simulink library "Teleop_lib"  (R2023b)
settings: Solver=VariableStepAuto  StartTime=0.0  StopTime=10.0  RelTol=1e-3
undefined symbols (not defined in the file): Spline_Num_Poses_default, Spline_Ref_Poses_default, TEST_Swerve_Mode_Override_Flag, TEST_Swerve_Mode_Steering, TEST_Swerve_Mode_Translation
settings Model: Creator=FIRSTMentor  LastModifiedBy=ander

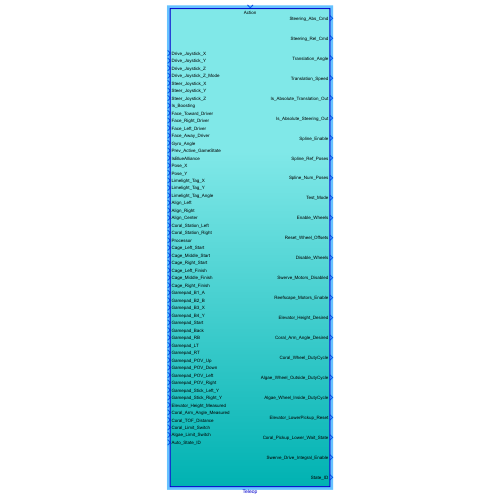
[thumbnail: Simulink's stored preview of the top-level diagram]
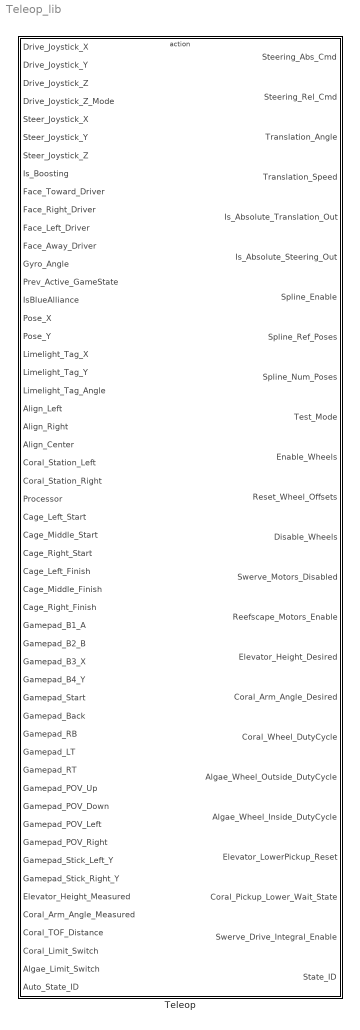
== system Teleop_lib ==
  Teleop : Subsystem  TreatAsAtomicUnit=on

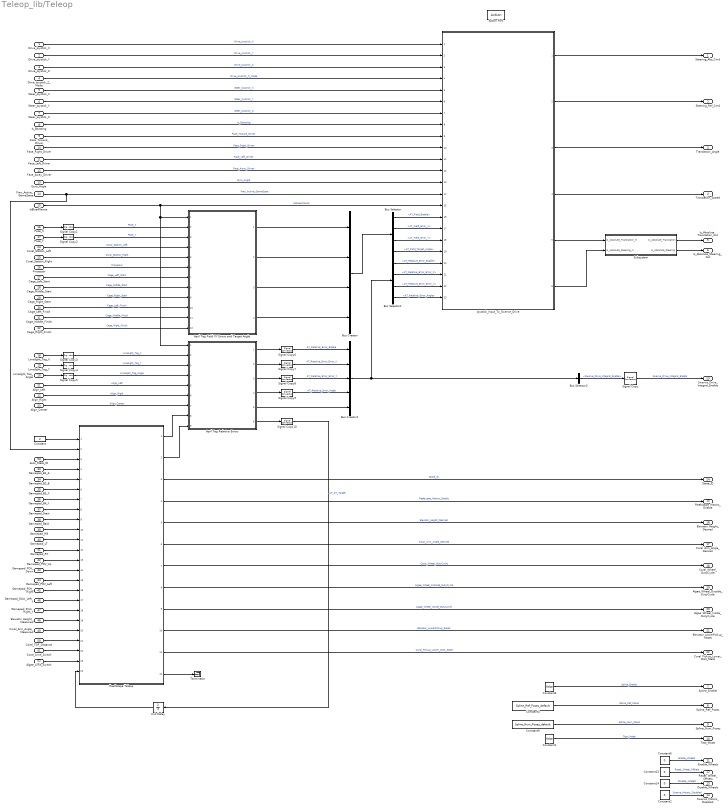
== system Teleop_lib/Teleop ==
  Drive_Joystick_X : Inport
  Drive_Joystick_Y : Inport  Port=2
  Drive_Joystick_Z : Inport  Port=3
  Drive_Joystick_Z_Mode : Inport  Port=4
  Steer_Joystick_X : Inport  Port=5
  Steer_Joystick_Y : Inport  Port=6
  Steer_Joystick_Z : Inport  Port=7
  Is_Boosting : Inport  Port=8
  Face_Toward_Driver : Inport  Port=9
  Face_Right_Driver : Inport  Port=10
  Face_Left_Driver : Inport  Port=11
  Face_Away_Driver : Inport  Port=12
  Gyro_Angle : Inport  Port=13
  Prev_Active_GameState : Inport  Port=14
  IsBlueAlliance : Inport  Port=15
  Pose_X : Inport  Port=16
  Pose_Y : Inport  Port=17
  Limelight_Tag_X : Inport  Port=18
  Limelight_Tag_Y : Inport  Port=19
  Limelight_Tag_Angle : Inport  Port=20
  Align_Left : Inport  Port=21
  Align_Right : Inport  Port=22
  Align_Center : Inport  Port=23
  Coral_Station_Left : Inport  Port=24
  Coral_Station_Right : Inport  Port=25
  Processor : Inport  Port=26
  Cage_Left_Start : Inport  Port=27
  Cage_Middle_Start : Inport  Port=28
  Cage_Right_Start : Inport  Port=29
  Cage_Left_Finish : Inport  Port=30
  Cage_Middle_Finish : Inport  Port=31
  Cage_Right_Finish : Inport  Port=32
  Gamepad_B1_A : Inport  Port=33
  Gamepad_B2_B : Inport  Port=34
  Gamepad_B3_X : Inport  Port=35
  Gamepad_B4_Y : Inport  Port=36
  Gamepad_Start : Inport  Port=37
  Gamepad_Back : Inport  Port=38
  Gamepad_RB : Inport  Port=39
  Gamepad_LT : Inport  Port=40
  Gamepad_RT : Inport  Port=41
  Gamepad_POV_Up : Inport  Port=42
  Gamepad_POV_Down : Inport  Port=43
  Gamepad_POV_Left : Inport  Port=44
  Gamepad_POV_Right : Inport  Port=45
  Gamepad_Stick_Left_Y : Inport  Port=46
  Gamepad_Stick_Right_Y : Inport  Port=47
  Elevator_Height_Measured : Inport  Port=48
  Coral_Arm_Angle_Measured : Inport  Port=49
  Coral_TOF_Distance : Inport  Port=50
  Coral_Limit_Switch : Inport  Port=51
  Algae_Limit_Switch : Inport  Port=52
  Auto_State_ID : Inport  Port=53
  Action Port : ActionPort  InitializeStates=reset
  April Tag Field XY Errors and Target Angle : Subsystem  ReferencedSubsystem=April_Tag_Field_Errors
  April Tag Relative Errors : Subsystem  ReferencedSubsystem=April_Tag_Relative_Errors
  Bus Creator : BusCreator  Inputs=4
  Bus Creator1 : BusCreator  Inputs=5
  Bus Selector : BusSelector  OutputSignals=AT_Field_Enable,AT_Field_Error_X,AT_Field_Error_Y,AT_Field_Target_Angle
  Bus Selector1 : BusSelector  OutputSignals=AT_Relative_Error_Enable,AT_Relative_Error_Error_X,AT_Relative_Error_Error_Y,AT_Relative_Error_Angle
  Bus Selector2 : BusSelector  OutputSignals=Swerve_Drive_Integral_Enable
  Constant : Constant  Value=2  OutDataTypeStr=uint8
  Constant1 : Constant  Value=false  OutDataTypeStr=boolean
  Constant13 : Constant  Value=0
  Constant14 : Constant  Value=0
  Constant2 : Constant  Value=0  OutDataTypeStr=boolean
  Constant3 : Constant  Value=false  OutDataTypeStr=boolean
  Constant4 : Constant  Value=Spline_Ref_Poses_default
  Constant6 : Constant  Value=0
  Constant9 : Constant  Value=Spline_Num_Poses_default  OutDataTypeStr=double
  Joystick_Input_To_Swerve_Drive : Subsystem  ReferencedSubsystem=Joystick_Input_To_Swerve_Drive_sub
  Reefscape Teleop : Subsystem  ReferencedSubsystem=Reefscape_Teleop_sub
  Signal Copy{,1..10} (11 alike) : SignalConversion  OverrideOpt=off
  Subsystem : Subsystem
  Terminator : Terminator
  Unit Delay : UnitDelay  SampleTime=-1  HasFrameUpgradeWarning=on
  Steering_Abs_Cmd : Outport
  Steering_Rel_Cmd : Outport  Port=2
  Translation_Angle : Outport  Port=3
  Translation_Speed : Outport  Port=4
  Is_Absolute_Translation_Out : Outport  Port=5
  Is_Absolute_Steering_Out : Outport  Port=6
  Spline_Enable : Outport  Port=7
  Spline_Ref_Poses : Outport  Port=8
  Spline_Num_Poses : Outport  Port=9
  Test_Mode : Outport  Port=10
  Enable_Wheels : Outport  Port=11
  Reset_Wheel_Offsets : Outport  Port=12
  Disable_Wheels : Outport  Port=13
  Swerve_Motors_Disabled : Outport  Port=14
  Reefscape_Motors_Enable : Outport  Port=15
  Elevator_Height_Desired : Outport  Port=16
  Coral_Arm_Angle_Desired : Outport  Port=17
  Coral_Wheel_DutyCycle : Outport  Port=18
  Algae_Wheel_Outside_DutyCycle : Outport  Port=19
  Algae_Wheel_Inside_DutyCycle : Outport  Port=20
  Elevator_LowerPickup_Reset : Outport  Port=21
  Coral_Pickup_Lower_Wait_State : Outport  Port=22
  Swerve_Drive_Integral_Enable : Outport  Port=23
  State_ID : Outport  Port=24
  wires:
  Signal Copy/1 -> Swerve_Drive_Integral_Enable/1  "Swerve_Drive_Integral_Enable"
  Steer_Joystick_X/1 -> Joystick_Input_To_Swerve_Drive/5  "Steer_Joystick_X"
  Steer_Joystick_Y/1 -> Joystick_Input_To_Swerve_Drive/6  "Steer_Joystick_Y"
  Drive_Joystick_X/1 -> Joystick_Input_To_Swerve_Drive/1  "Drive_Joystick_X"
  Drive_Joystick_Y/1 -> Joystick_Input_To_Swerve_Drive/2  "Drive_Joystick_Y"
  Joystick_Input_To_Swerve_Drive/1 -> Steering_Abs_Cmd/1
  Joystick_Input_To_Swerve_Drive/2 -> Steering_Rel_Cmd/1
  Joystick_Input_To_Swerve_Drive/3 -> Translation_Angle/1
  Joystick_Input_To_Swerve_Drive/4 -> Translation_Speed/1
  Is_Boosting/1 -> Joystick_Input_To_Swerve_Drive/8  "Is_Boosting"
  Constant9/1 -> Spline_Num_Poses/1  "Spline_Num_Poses"
  Constant4/1 -> Spline_Ref_Poses/1  "Spline_Ref_Poses"
  Constant3/1 -> Spline_Enable/1  "Spline_Enable"
  Constant1/1 -> Test_Mode/1  "Test_Mode"
  Drive_Joystick_Z/1 -> Joystick_Input_To_Swerve_Drive/3  "Drive_Joystick_Z"
  Steer_Joystick_Z/1 -> Joystick_Input_To_Swerve_Drive/7  "Steer_Joystick_Z"
  Face_Toward_Driver/1 -> Joystick_Input_To_Swerve_Drive/9  "Face_Toward_Driver"
  Face_Right_Driver/1 -> Joystick_Input_To_Swerve_Drive/10  "Face_Right_Driver"
  Face_Left_Driver/1 -> Joystick_Input_To_Swerve_Drive/11  "Face_Left_Driver"
  Face_Away_Driver/1 -> Joystick_Input_To_Swerve_Drive/12  "Face_Away_Driver"
  Pose_X/1 -> Signal Copy1/1
  Pose_Y/1 -> Signal Copy2/1
  IsBlueAlliance/1 -> Joystick_Input_To_Swerve_Drive/15, April Tag Relative Errors/1, April Tag Field XY Errors and Target Angle/1  "IsBlueAlliance"
  Drive_Joystick_Z_Mode/1 -> Joystick_Input_To_Swerve_Drive/4  "Drive_Joystick_Z_Mode"
  Gyro_Angle/1 -> Joystick_Input_To_Swerve_Drive/13  "Gyro_Angle"
  Align_Left/1 -> April Tag Relative Errors/5  "Align_Left"
  Align_Right/1 -> April Tag Relative Errors/6  "Align_Right"
  Align_Center/1 -> April Tag Relative Errors/7  "Align_Center"
  Limelight_Tag_X/1 -> Signal Copy3/1
  Limelight_Tag_Y/1 -> Signal Copy4/1
  Limelight_Tag_Angle/1 -> Signal Copy5/1
  Constant13/1 -> Reset_Wheel_Offsets/1  "Reset_Wheel_Offsets"
  Constant14/1 -> Disable_Wheels/1  "Disable_Wheels"
  Prev_Active_GameState/1 -> Joystick_Input_To_Swerve_Drive/14, Reefscape Teleop/2  "Prev_Active_GameState"
  Constant2/1 -> Swerve_Motors_Disabled/1  "Swerve_Motors_Disabled"
  Constant6/1 -> Enable_Wheels/1  "Enable_Wheels"
  Signal Copy3/1 -> April Tag Relative Errors/2  "Limelight_Tag_X"
  Signal Copy4/1 -> April Tag Relative Errors/3  "Limelight_Tag_Y"
  Signal Copy5/1 -> April Tag Relative Errors/4  "Limelight_Tag_Angle"
  Coral_Station_Left/1 -> April Tag Field XY Errors and Target Angle/4  "Coral_Station_Left"
  Coral_Station_Right/1 -> April Tag Field XY Errors and Target Angle/5  "Coral_Station_Right"
  Processor/1 -> April Tag Field XY Errors and Target Angle/6  "Processor"
  Signal Copy1/1 -> April Tag Field XY Errors and Target Angle/2  "Pose_X"
  Signal Copy2/1 -> April Tag Field XY Errors and Target Angle/3  "Pose_Y"
  Joystick_Input_To_Swerve_Drive/5 -> Subsystem/1(Is_Absolute_Translation_In)
  Joystick_Input_To_Swerve_Drive/6 -> Subsystem/2(Is_Absolute_Steering_In)
  Subsystem/1(Is_Absolute_Translation) -> Is_Absolute_Translation_Out/1
  Subsystem/2(Is_Absolute_Steering) -> Is_Absolute_Steering_Out/1
  Reefscape Teleop/1 -> April Tag Relative Errors/8
  April Tag Field XY Errors and Target Angle/1 -> Bus Creator/1
  April Tag Field XY Errors and Target Angle/2 -> Bus Creator/2
  April Tag Field XY Errors and Target Angle/3 -> Bus Creator/3
  April Tag Field XY Errors and Target Angle/4 -> Bus Creator/4
  April Tag Relative Errors/1 -> Signal Copy6/1
  April Tag Relative Errors/2 -> Signal Copy7/1
  April Tag Relative Errors/3 -> Signal Copy8/1
  April Tag Relative Errors/4 -> Signal Copy9/1
  Bus Creator/1 -> Bus Selector/1
  Bus Selector/1 -> Joystick_Input_To_Swerve_Drive/16  "<AT_Field_Enable>"
  Bus Selector/2 -> Joystick_Input_To_Swerve_Drive/17  "<AT_Field_Error_X>"
  Bus Selector/3 -> Joystick_Input_To_Swerve_Drive/18  "<AT_Field_Error_Y>"
  Bus Selector/4 -> Joystick_Input_To_Swerve_Drive/19  "<AT_Field_Target_Angle>"
  Bus Creator1/1 -> Bus Selector2/1, Bus Selector1/1
  Bus Selector1/1 -> Joystick_Input_To_Swerve_Drive/20  "<AT_Relative_Error_Enable>"
  Bus Selector1/2 -> Joystick_Input_To_Swerve_Drive/21  "<AT_Relative_Error_Error_X>"
  Bus Selector1/3 -> Joystick_Input_To_Swerve_Drive/22  "<AT_Relative_Error_Error_Y>"
  Bus Selector1/4 -> Joystick_Input_To_Swerve_Drive/23  "<AT_Relative_Error_Angle>"
  Cage_Left_Start/1 -> April Tag Field XY Errors and Target Angle/7  "Cage_Left_Start"
  Cage_Middle_Start/1 -> April Tag Field XY Errors and Target Angle/8  "Cage_Middle_Start"
  Cage_Right_Start/1 -> April Tag Field XY Errors and Target Angle/9  "Cage_Right_Start"
  Cage_Left_Finish/1 -> April Tag Field XY Errors and Target Angle/10  "Cage_Left_Finish"
  Cage_Middle_Finish/1 -> April Tag Field XY Errors and Target Angle/11  "Cage_Middle_Finish"
  Cage_Right_Finish/1 -> April Tag Field XY Errors and Target Angle/12  "Cage_Right_Finish"
  Reefscape Teleop/2 -> April Tag Relative Errors/9
  Reefscape Teleop/4 -> Reefscape_Motors_Enable/1  "Reefscape_Motors_Enable"
  Reefscape Teleop/5 -> Elevator_Height_Desired/1  "Elevator_Height_Desired"
  Reefscape Teleop/6 -> Coral_Arm_Angle_Desired/1  "Coral_Arm_Angle_Desired"
  Reefscape Teleop/7 -> Coral_Wheel_DutyCycle/1  "Coral_Wheel_DutyCycle"
  Reefscape Teleop/8 -> Algae_Wheel_Outside_DutyCycle/1  "Algae_Wheel_Outside_DutyCycle"
  Reefscape Teleop/9 -> Algae_Wheel_Inside_DutyCycle/1  "Algae_Wheel_Inside_DutyCycle"
  Reefscape Teleop/10 -> Elevator_LowerPickup_Reset/1  "Elevator_LowerPickup_Reset"
  Reefscape Teleop/11 -> Coral_Pickup_Lower_Wait_State/1  "Coral_Pickup_Lower_Wait_State"
  April Tag Relative Errors/5 -> Bus Creator1/5
  Bus Selector2/1 -> Signal Copy/1  "<Swerve_Drive_Integral_Enable>"
  April Tag Relative Errors/6 -> Signal Copy10/1
  Reefscape Teleop/12 -> Terminator/1
  Unit Delay/1 -> Reefscape Teleop/24
  Constant/1 -> Reefscape Teleop/1
  Auto_State_ID/1 -> Reefscape Teleop/3
  Gamepad_B1_A/1 -> Reefscape Teleop/4
  Gamepad_B2_B/1 -> Reefscape Teleop/5
  Gamepad_B3_X/1 -> Reefscape Teleop/6
  Gamepad_B4_Y/1 -> Reefscape Teleop/7
  Gamepad_Start/1 -> Reefscape Teleop/8
  Gamepad_Back/1 -> Reefscape Teleop/9
  Gamepad_RB/1 -> Reefscape Teleop/10
  Gamepad_LT/1 -> Reefscape Teleop/11
  Gamepad_RT/1 -> Reefscape Teleop/12
  Gamepad_POV_Up/1 -> Reefscape Teleop/13
  Gamepad_POV_Down/1 -> Reefscape Teleop/14
  Gamepad_POV_Left/1 -> Reefscape Teleop/15
  Gamepad_POV_Right/1 -> Reefscape Teleop/16
  Gamepad_Stick_Left_Y/1 -> Reefscape Teleop/17
  Gamepad_Stick_Right_Y/1 -> Reefscape Teleop/18
  Elevator_Height_Measured/1 -> Reefscape Teleop/19
  Coral_Arm_Angle_Measured/1 -> Reefscape Teleop/20
  Coral_TOF_Distance/1 -> Reefscape Teleop/21
  Coral_Limit_Switch/1 -> Reefscape Teleop/22
  Algae_Limit_Switch/1 -> Reefscape Teleop/23
  Reefscape Teleop/3 -> State_ID/1  "State_ID"
  Signal Copy6/1 -> Bus Creator1/1  "AT_Relative_Error_Enable"
  Signal Copy7/1 -> Bus Creator1/2  "AT_Relative_Error_Error_X"
  Signal Copy8/1 -> Bus Creator1/3  "AT_Relative_Error_Error_Y"
  Signal Copy9/1 -> Bus Creator1/4  "AT_Relative_Error_Angle"
  Signal Copy10/1 -> Unit Delay/1  "AT_On_Target"

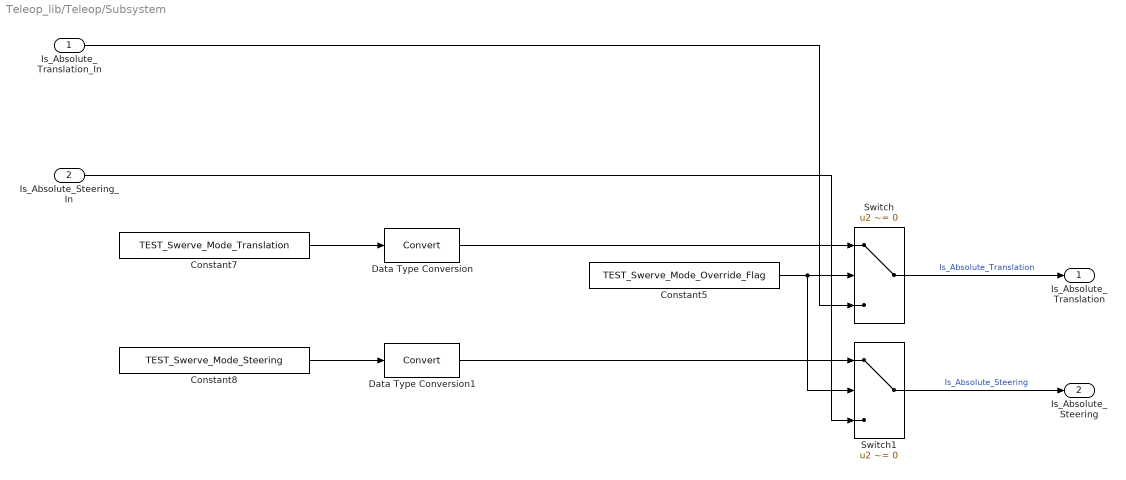
== system Teleop_lib/Teleop/Subsystem ==
  Is_Absolute_Translation_In : Inport
  Is_Absolute_Steering_In : Inport  Port=2
  Constant5 : Constant  Value=TEST_Swerve_Mode_Override_Flag
  Constant7 : Constant  Value=TEST_Swerve_Mode_Translation
  Constant8 : Constant  Value=TEST_Swerve_Mode_Steering
  Data Type Conversion : DataTypeConversion  SaturateOnIntegerOverflow=off  RndMeth=Floor
  Data Type Conversion1 : DataTypeConversion  SaturateOnIntegerOverflow=off  RndMeth=Floor
  Switch : Switch  Criteria=u2 ~= 0  SaturateOnIntegerOverflow=off  InputSameDT=off
  Switch1 : Switch  Criteria=u2 ~= 0  SaturateOnIntegerOverflow=off  InputSameDT=off
  Is_Absolute_Translation : Outport
  Is_Absolute_Steering : Outport  Port=2
  wires:
  Constant5/1 -> Switch/2, Switch1/2
  Data Type Conversion/1 -> Switch/1
  Data Type Conversion1/1 -> Switch1/1
  Is_Absolute_Translation_In/1 -> Switch/3
  Switch/1 -> Is_Absolute_Translation/1  "Is_Absolute_Translation"
  Constant8/1 -> Data Type Conversion1/1
  Constant7/1 -> Data Type Conversion/1
  Is_Absolute_Steering_In/1 -> Switch1/3
  Switch1/1 -> Is_Absolute_Steering/1  "Is_Absolute_Steering"
